simulink model "edmsrc8"  (R2019a)
settings: Solver=ode23t  StartTime=0.0  StopTime=0.001  MaxStep=1e-6  MinStep=1e-7  RelTol=1e-3  EnableMultiTasking=on
values from neighbouring files (symbols this model uses):
  Iref = 5    [setpara1.m]
  Vref = 70    [setpara1.m]
libraries: powerlib x12
settings Model: Creator=FC Lab  LastModifiedBy=Prakhar
settings DataIOCC: LimitDataPoints=on  ReturnWorkspaceOutputs=off
settings OptimizationCC: LifeSpan=inf
settings DebuggingCC: AllowSymbolicDim=off  SFUnexpectedBacktrackingDiag=warning  SFNoUnconditionalDefaultTransitionDiag=warning  SFExecutionAtInitializationDiag=none  ArithmeticOperatorsInVariantConditions=warning
settings ModelReferenceCC: PropagateSignalLabelsOutOfModel=off
settings SFSimCC: SimUseLocalCustomCode=off
settings RTWCC: RTWUseLocalCustomCode=off
settings CodeAppCC: StateflowObjectComments=on
settings GRTTargetCC: TargetLangStandard=C89/C90 (ANSI)
settings ConfigComp: CovMetricSettings=dw  CovHtmlReporting=on  CovSaveCumulativeToWorkspaceVar=on  CovSaveSingleToWorkspaceVar=on  CovExternalEMLEnable=off
settings SimscapeCC: SimscapeNormalizeSystem=off

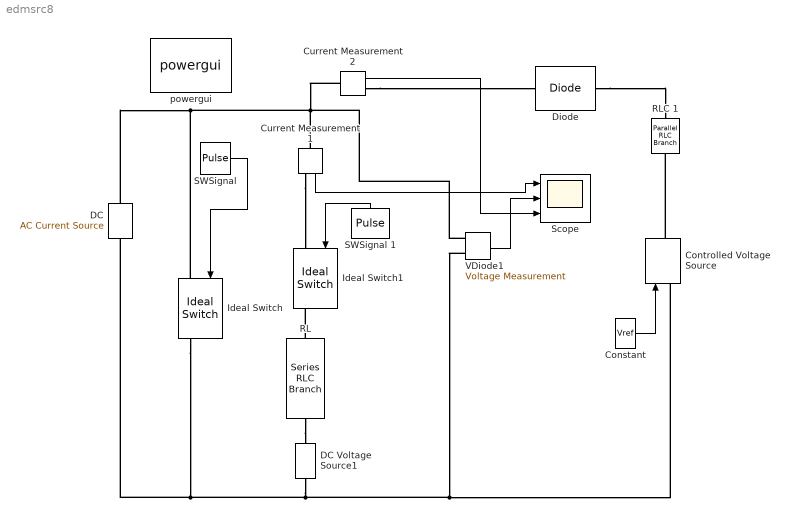
== system edmsrc8 ==
  " RLC 1" : powerlib/Elements/Parallel RLC Branch  LConnTagsString=a  RConnTagsString=__new0  BranchType=R  Resistance=0.001  Inductance=1e-3  SetiL0=off  InitialCurrent=0  Capacitance=0.3e-6  Setx0=off  InitialVoltage=0  Measurements=None
      settings: SourceProductName=Simscape Electrical
  Constant : Constant  Value=Vref
  Controlled Voltage Source : powerlib/Electrical Sources/Controlled Voltage Source  Initialize=on  Source_Type=DC  Amplitude=Vref  Phase=0  Frequency=0  Measurements=None
      settings: SourceProductName=Simscape Electrical
  Current Measurement1 : powerlib/Measurements/Current Measurement  PhasorSimulation=off  OutputType=Complex  PSBequivalent=0
      settings: SourceProductName=Simscape Electrical
  Current Measurement2 : powerlib/Measurements/Current Measurement  PhasorSimulation=off  OutputType=Complex  PSBequivalent=0
      settings: SourceProductName=Simscape Electrical
  "DC " : powerlib/Electrical Sources/AC Current Source  Amplitude=Iref  Phase=90  Frequency=0  SampleTime=0  Measurements=None
      settings: SourceProductName=Simscape Electrical  SourceProductBaseCode=PS
  DC Voltage Source1 : powerlib/Electrical Sources/DC Voltage Source  Amplitude=40  Measurements=Voltage
      settings: SourceProductName=Simscape Electrical
  Diode : powerlib/Power Electronics/Diode  Ron=0.001  Lon=0  Vf=0.8  IC=0  UseSnubber=off  Rs=500  Cs=250e-9  Measurements=off
      settings: SourceProductName=Simscape Electrical
  Ideal Switch : powerlib/Power Electronics/Ideal Switch  Ron=0.001  Lon=0  IC=0  Rs=1e5  Cs=inf  Measurements=on
      settings: SourceProductName=Simscape Electrical
  Ideal Switch1 : powerlib/Power Electronics/Ideal Switch  Ron=0.001  Lon=0  IC=0  Rs=1e5  Cs=inf  Measurements=on
      settings: SourceProductName=Simscape Electrical
  RL : powerlib/Elements/Series RLC Branch  LConnTagsString=__new0  RConnTagsString=__new0  BranchType=R  Resistance=1  Inductance=3e-6  SetiL0=off  InitialCurrent=0  Capacitance=1e-6  Setx0=off  InitialVoltage=0  Measurements=None
      settings: SourceProductName=Simscape Electrical
  "SWSignal " : DiscretePulseGenerator  PulseType=Time based  Period=100e-6  PulseWidth=80  PhaseDelay=20e-6
  SWSignal 1 : DiscretePulseGenerator  PulseType=Time based  Period=100e-6  PulseWidth=15  PhaseDelay=5e-6
  Scope : Scope  NumInputPorts=3
  VDiode1 : powerlib/Measurements/Voltage Measurement  PhasorSimulation=off  OutputType=Complex  PSBequivalent=0
      settings: SourceProductName=Simscape Electrical
  powergui : powerlib/powergui  Priority=1  SimulationMode=Continuous  SampleTime=5e-07  frequency=60  Iterations=50  frequencyindice=0  Pbase=100e6  ErrMax=1e-4  UnitsV=kV  UnitsW=MW  buscounter=0  FunctionMessages=off  echomessages=off  EnableUseOfTLC=off  CurrentSourceSwitches=off  DisableSnubberDevices=off  DisableRonSwitches=off  DisableVfSwitches=off  DisplayEquations=off  AutomaticDiscreteSolvers=off  SolverType=Backward Euler  Interpol=off  ExternalGateDelay=off  methode=off  Ts=0  x0status=zero  SPID=on  SwTol=0  HookPort=off  NonlinearTolerance=0  nMaxIteration=15  ContinueOnMaxIteration=off  RestoreLinks=warning  ResistiveCurrentMeasurement=off  Frange=[0:2:500]  Ylog=off  Xlog=on  ShowGrid=off  save=off  variable=ZData  structure=ScopeData  ZoomFFT=off  StartTime=0.0  cycles=5  DisplayStyle=2  fundamental=50  FreqAxis=off  MaxFrequency=50000  frequencyindicesteady=1  RmsSteady=1  display=off
      settings: SourceProductName=Simscape Electrical
  wires:
  "SWSignal "/1 -> Ideal Switch/1
  SWSignal 1/1 -> Ideal Switch1/1
  Current Measurement1/1 -> Scope/1
  VDiode1/1 -> Scope/2
  Constant/1 -> Controlled Voltage Source/1
  Current Measurement2/1 -> Scope/3
  connections:
  "DC "/RConn1 -- VDiode1/LConn1 -- Current Measurement2/LConn1 -- Current Measurement1/LConn1 -- Ideal Switch/LConn1
  VDiode1/LConn2 -- Controlled Voltage Source/LConn1 -- DC Voltage Source1/LConn1 -- Ideal Switch/RConn1 -- "DC "/LConn1
  Current Measurement1/RConn1 -- Ideal Switch1/LConn1
  Diode/RConn1 -- " RLC 1"/LConn1
  Controlled Voltage Source/RConn1 -- " RLC 1"/RConn1
  Current Measurement2/RConn1 -- Diode/LConn1
  RL/LConn1 -- Ideal Switch1/RConn1
  RL/RConn1 -- DC Voltage Source1/RConn1
